simulink library "LIB_TF_G_112"  (Simulink 8.6)
settings: Solver=ode45  StartTime=0.0  StopTime=10.0  RelTol=1e-3
PreLoadFcn:
  | if exist('tl_preloadfcn','file'), tl_preloadfcn(gcs,402); end
PostLoadFcn:
  | if exist('tl_postloadfcn','file'), tl_postloadfcn(gcs,402); end
undefined symbols (not defined in the file): ddv, u2, u3
libraries: tllib x3
(part 1 of 4)
CloseFcn:
  | if exist('tl_closefcn','file'), tl_closefcn(gcs); end
settings Model: TLRevision=402  Creator=cedric.sauvage  LastModifiedBy=audrey.vache

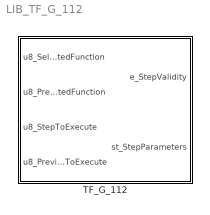
== system LIB_TF_G_112 ==
  TF_G_112 : Subsystem  TreatAsAtomicUnit=on

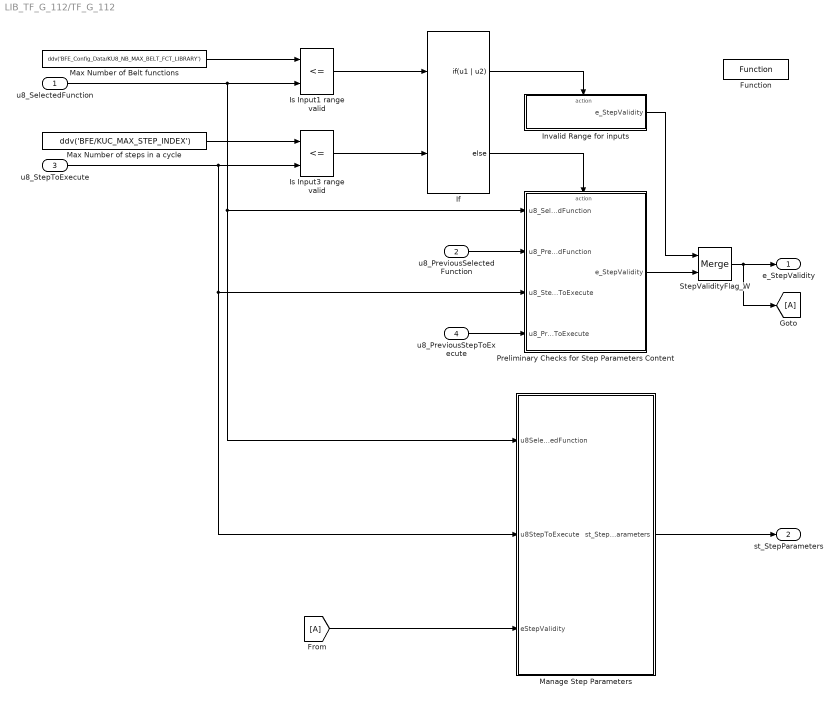
== system LIB_TF_G_112/TF_G_112 ==
  u8_SelectedFunction : Inport
  u8_PreviousSelectedFunction : Inport  Port=2
  u8_StepToExecute : Inport  Port=3
  u8_PreviousStepToExecute : Inport  Port=4
  Function : tllib/Function  data={'stepfunctionname','M_StepPreprocessing','stepfunctionclass','STATIC_FCN_ASR4','date',736467.70272937499}  displayString=FUNCTION
  If : If  NumInputs=2  IfExpression=u1 | u2
  Invalid Range for inputs : Subsystem  TreatAsAtomicUnit=on
  Is Input1 range valid : RelationalOperator  Operator=<=  OutDataTypeStr=boolean  mask(TL_RelationalOperator){data={'date',735951.66829449078}}
      settings: DeleteFcn=if exist('delete_tlblock','file')==2,delete_tlblock(gcbh);end  NameChangeFcn=if exist('rename_tlblock','file')==2,rename_tlblock(gcbh);end  OpenFcn=if exist('tl_open_blockdlg','file')==2,tl_open_blockdlg(gcbh);else,open_system(gcbh,'parameter');end
      mask Help: eval(['if exist(''tl_online_help'',''file'') == 2, tl_online_help(''Topic'',''TL_RelationalOperator''),else, web([''jar:file:///'',matlabroot,''/help/toolbox/simulink/help.jar!/slref/' lower(get_param(gcbh,'Blocktype')) '.html''], ''-helpbrowser''),end'])
      mask Display: plot([-0.05, 1.05, NaN, -0.05, 1.05],[.01, .01, NaN, .99, .99])
  Is Input3 range valid : RelationalOperator  Operator=<=  OutDataTypeStr=boolean  mask(TL_RelationalOperator){data={'date',735951.66829423606}}
      settings: DeleteFcn=if exist('delete_tlblock','file')==2,delete_tlblock(gcbh);end  NameChangeFcn=if exist('rename_tlblock','file')==2,rename_tlblock(gcbh);end  OpenFcn=if exist('tl_open_blockdlg','file')==2,tl_open_blockdlg(gcbh);else,open_system(gcbh,'parameter');end
      mask Help: eval(['if exist(''tl_online_help'',''file'') == 2, tl_online_help(''Topic'',''TL_RelationalOperator''),else, web([''jar:file:///'',matlabroot,''/help/toolbox/simulink/help.jar!/slref/' lower(get_param(gcbh,'Blocktype')) '.html''], ''-helpbrowser''),end'])
      mask Display: plot([-0.05, 1.05, NaN, -0.05, 1.05],[.01, .01, NaN, .99, .99])
  Manage Step Parameters : Subsystem  TreatAsAtomicUnit=on
  Max Number of Belt functions : Constant  Value=ddv('BFE_Config_Data/KU8_NB_MAX_BELT_FCT_LIBRARY')  mask(TL_Constant){data={'output',{'variable','BFE_Config_Data/KU8_NB_MAX_BELT_FCT_LIBRARY'},'date',735951.66825344902}}
      settings: CopyFcn=if exist('tl_reset_reviewflag','file')==2,tl_reset_reviewflag(gcbh);end  DeleteFcn=if exist('delete_tlblock','file')==2,delete_tlblock(gcbh);end  NameChangeFcn=if exist('rename_tlblock','file')==2,rename_tlblock(gcbh);end  OpenFcn=if exist('tl_open_blockdlg','file')==2,tl_open_blockdlg(gcbh);else,open_system(gcbh,'parameter');end
      mask Help: eval(['if exist(''tl_online_help'',''file'') == 2, tl_online_help(''Topic'',''TL_Constant''),else, web([''jar:file:///'',matlabroot,''/help/toolbox/simulink/help.jar!/slref/' lower(get_param(gcbh,'Blocktype')) '.html''], ''-helpbrowser''),end'])
      mask Display: plot([-0.05, 1.05, NaN, -0.05, 1.05],[.01, .01, NaN, .99, .99])
  Max Number of steps in a cycle : Constant  Value=ddv('BFE/KUC_MAX_STEP_INDEX')  mask(TL_Constant){data={'output',{'variable','BFE/KUC_MAX_STEP_INDEX'},'date',735951.66825306718}}
      settings: CopyFcn=if exist('tl_reset_reviewflag','file')==2,tl_reset_reviewflag(gcbh);end  DeleteFcn=if exist('delete_tlblock','file')==2,delete_tlblock(gcbh);end  NameChangeFcn=if exist('rename_tlblock','file')==2,rename_tlblock(gcbh);end  OpenFcn=if exist('tl_open_blockdlg','file')==2,tl_open_blockdlg(gcbh);else,open_system(gcbh,'parameter');end
      mask Help: eval(['if exist(''tl_online_help'',''file'') == 2, tl_online_help(''Topic'',''TL_Constant''),else, web([''jar:file:///'',matlabroot,''/help/toolbox/simulink/help.jar!/slref/' lower(get_param(gcbh,'Blocktype')) '.html''], ''-helpbrowser''),end'])
      mask Display: plot([-0.05, 1.05, NaN, -0.05, 1.05],[.01, .01, NaN, .99, .99])
  Preliminary Checks for Step Parameters Content : Subsystem  TreatAsAtomicUnit=on
  StepValidityFlag_W : Merge  InitialOutput=0  mask(TL_Merge){data={'logdata',{'maxnumvals',2500,'loggingmode',1},'output',{'name','eStepValidity','type','UInt8','inheritscaling',0},'date',735951.66823748848}}
      settings: CopyFcn=if exist('tl_reset_reviewflag','file')==2,tl_reset_reviewflag(gcbh);end  DeleteFcn=if exist('delete_tlblock','file')==2,delete_tlblock(gcbh);end  NameChangeFcn=if exist('rename_tlblock','file')==2,rename_tlblock(gcbh);end  OpenFcn=if exist('tl_open_blockdlg','file')==2,tl_open_blockdlg(gcbh);else,open_system(gcbh,'parameter');end
      mask Help: eval(['if exist(''tl_online_help'',''file'') == 2, tl_online_help(''Topic'',''TL_Merge''),else, web([''jar:file:///'',matlabroot,''/help/toolbox/simulink/help.jar!/slref/' lower(get_param(gcbh,'Blocktype')) '.html''], ''-helpbrowser''),end'])
      mask Display: plot([-0.05, 1.05, NaN, -0.05, 1.05],[.01, .01, NaN, .99, .99])
  e_StepValidity : Outport
  st_StepParameters : Outport  Port=2  OutDataTypeStr=Bus: stStepParameters
  wires:
  u8_SelectedFunction/1 -> Is Input1 range valid/2, Preliminary Checks for Step Parameters Content/1(u8_SelectedFunction), Manage Step Parameters/1(u8SelectedFunction)
  Max Number of Belt functions/1 -> Is Input1 range valid/1
  Max Number of steps in a cycle/1 -> Is Input3 range valid/1
  u8_StepToExecute/1 -> Is Input3 range valid/2, Preliminary Checks for Step Parameters Content/3(u8_StepToExecute), Manage Step Parameters/2(u8StepToExecute)
  If/1 -> Invalid Range for inputs/Action
  Is Input1 range valid/1 -> If/1
  Is Input3 range valid/1 -> If/2
  If/2 -> Preliminary Checks for Step Parameters Content/Action
  u8_PreviousSelectedFunction/1 -> Preliminary Checks for Step Parameters Content/2(u8_PreviousSelectedFunction)
  u8_PreviousStepToExecute/1 -> Preliminary Checks for Step Parameters Content/4(u8_PreviousStepToExecute)
  Preliminary Checks for Step Parameters Content/1(e_StepValidity) -> StepValidityFlag_W/2
  Invalid Range for inputs/1(e_StepValidity) -> StepValidityFlag_W/1
  StepValidityFlag_W/1 -> e_StepValidity/1, [A]
  Manage Step Parameters/1(st_StepParameters) -> st_StepParameters/1
  [A] -> Manage Step Parameters/3(eStepValidity)

== system LIB_TF_G_112/TF_G_112/Invalid Range for inputs ==
  note: COVERS: DES_TF_G_915
      | COVERS: DES_TF_G_916
      | COVERS: DES_TF_G_922
      | COVERS: DES_TF_G_923
  Action Port : ActionPort
  Invalid Step Key Value : Constant  Value=ddv('Internal_Interfaces/Enumerated_values/Step_Validity/KE_INVALID_STEP')  mask(TL_Constant){data={'output',{'variable','Internal_Interfaces/Enumerated_values/Step_Validity/KE_INVALID_STEP'},'date',735951.66829484957}}
      settings: CopyFcn=if exist('tl_reset_reviewflag','file')==2,tl_reset_reviewflag(gcbh);end  DeleteFcn=if exist('delete_tlblock','file')==2,delete_tlblock(gcbh);end  NameChangeFcn=if exist('rename_tlblock','file')==2,rename_tlblock(gcbh);end  OpenFcn=if exist('tl_open_blockdlg','file')==2,tl_open_blockdlg(gcbh);else,open_system(gcbh,'parameter');end
      mask Help: eval(['if exist(''tl_online_help'',''file'') == 2, tl_online_help(''Topic'',''TL_Constant''),else, web([''jar:file:///'',matlabroot,''/help/toolbox/simulink/help.jar!/slref/' lower(get_param(gcbh,'Blocktype')) '.html''], ''-helpbrowser''),end'])
      mask Display: plot([-0.05, 1.05, NaN, -0.05, 1.05],[.01, .01, NaN, .99, .99])
  e_StepValidity : Outport  InitialOutput=0
  wires:
  Invalid Step Key Value/1 -> e_StepValidity/1

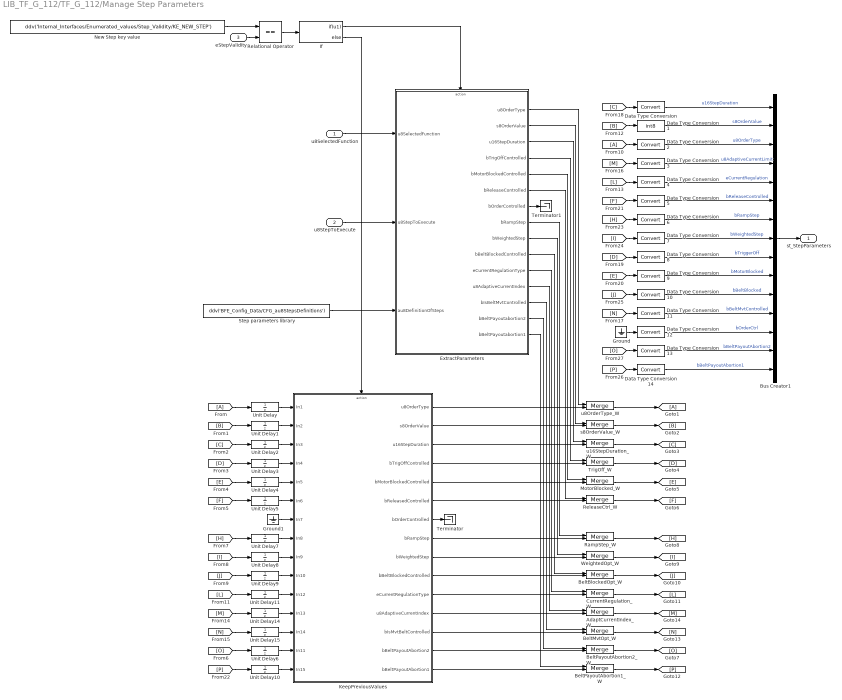
== system LIB_TF_G_112/TF_G_112/Manage Step Parameters ==
  u8SelectedFunction : Inport
  u8StepToExecute : Inport  Port=2
  eStepValidity : Inport  Port=3
  AdaptCurrentIndex_W : Merge  RequirementInfo={} %GIDa_e2928cb5_e14c_431e_87bc_c0c42f6fb32a  InitialOutput=ddv('Internal_Interfaces/stStepParameters/Components/u8AdaptCurrentLimit')  mask(TL_Merge){data={'logdata',{'loggingmode',1},'output',{'variable','Internal_Interfaces/stStepParameters/Components/u8AdaptCurrentLimit','inheritscaling',0},'date',735951.66829396994}}
      settings: CopyFcn=if exist('tl_reset_reviewflag','file')==2,tl_reset_reviewflag(gcbh);end  DeleteFcn=if exist('delete_tlblock','file')==2,delete_tlblock(gcbh);end  NameChangeFcn=if exist('rename_tlblock','file')==2,rename_tlblock(gcbh);end  OpenFcn=if exist('tl_open_blockdlg','file')==2,tl_open_blockdlg(gcbh);else,open_system(gcbh,'parameter');end
      mask Help: eval(['if exist(''tl_online_help'',''file'') == 2, tl_online_help(''Topic'',''TL_Merge''),else, web([''jar:file:///'',matlabroot,''/help/toolbox/simulink/help.jar!/slref/' lower(get_param(gcbh,'Blocktype')) '.html''], ''-helpbrowser''),end'])
      mask Display: plot([-0.05, 1.05, NaN, -0.05, 1.05],[.01, .01, NaN, .99, .99])
  BeltBlockedOpt_W : Merge  RequirementInfo={} %GIDa_0720534a_6e37_423d_8805_9648979410e2  InitialOutput=ddv('Internal_Interfaces/stStepParameters/Components/bBeltBlocked')  mask(TL_Merge){data={'logdata',{'loggingmode',1},'output',{'variable','Internal_Interfaces/stStepParameters/Components/bBeltBlocked','inheritscaling',0},'date',735951.66829357634}}
      settings: CopyFcn=if exist('tl_reset_reviewflag','file')==2,tl_reset_reviewflag(gcbh);end  DeleteFcn=if exist('delete_tlblock','file')==2,delete_tlblock(gcbh);end  NameChangeFcn=if exist('rename_tlblock','file')==2,rename_tlblock(gcbh);end  OpenFcn=if exist('tl_open_blockdlg','file')==2,tl_open_blockdlg(gcbh);else,open_system(gcbh,'parameter');end
      mask Help: eval(['if exist(''tl_online_help'',''file'') == 2, tl_online_help(''Topic'',''TL_Merge''),else, web([''jar:file:///'',matlabroot,''/help/toolbox/simulink/help.jar!/slref/' lower(get_param(gcbh,'Blocktype')) '.html''], ''-helpbrowser''),end'])
      mask Display: plot([-0.05, 1.05, NaN, -0.05, 1.05],[.01, .01, NaN, .99, .99])
  BeltMvtOpt_W : Merge  RequirementInfo={} %GIDa_23d3dad0_6239_4fa2_ab83_c69ad9dd92c5  InitialOutput=ddv('Internal_Interfaces/stStepParameters/Components/bBeltMvtDetection')  mask(TL_Merge){data={'logdata',{'loggingmode',1},'output',{'variable','Internal_Interfaces/stStepParameters/Components/bBeltMvtDetection','inheritscaling',0},'date',735951.66829317133}}
      settings: CopyFcn=if exist('tl_reset_reviewflag','file')==2,tl_reset_reviewflag(gcbh);end  DeleteFcn=if exist('delete_tlblock','file')==2,delete_tlblock(gcbh);end  NameChangeFcn=if exist('rename_tlblock','file')==2,rename_tlblock(gcbh);end  OpenFcn=if exist('tl_open_blockdlg','file')==2,tl_open_blockdlg(gcbh);else,open_system(gcbh,'parameter');end
      mask Help: eval(['if exist(''tl_online_help'',''file'') == 2, tl_online_help(''Topic'',''TL_Merge''),else, web([''jar:file:///'',matlabroot,''/help/toolbox/simulink/help.jar!/slref/' lower(get_param(gcbh,'Blocktype')) '.html''], ''-helpbrowser''),end'])
      mask Display: plot([-0.05, 1.05, NaN, -0.05, 1.05],[.01, .01, NaN, .99, .99])
  BeltPayoutAbortion1_W : Merge  RequirementInfo={} %GIDa_36c1306a_9619_4e1f_b53e_761d8c217ca4  InitialOutput=ddv('Internal_Interfaces/stStepParameters/Components/bBeltPayoutAbortion1')  mask(TL_Merge){data={'logdata',{'loggingmode',1},'output',{'variable','Internal_Interfaces/stStepParameters/Components/bBeltPayoutAbortion1','inheritscaling',0},'date',735951.66829277773}}
      settings: CopyFcn=if exist('tl_reset_reviewflag','file')==2,tl_reset_reviewflag(gcbh);end  DeleteFcn=if exist('delete_tlblock','file')==2,delete_tlblock(gcbh);end  NameChangeFcn=if exist('rename_tlblock','file')==2,rename_tlblock(gcbh);end  OpenFcn=if exist('tl_open_blockdlg','file')==2,tl_open_blockdlg(gcbh);else,open_system(gcbh,'parameter');end
      mask Help: eval(['if exist(''tl_online_help'',''file'') == 2, tl_online_help(''Topic'',''TL_Merge''),else, web([''jar:file:///'',matlabroot,''/help/toolbox/simulink/help.jar!/slref/' lower(get_param(gcbh,'Blocktype')) '.html''], ''-helpbrowser''),end'])
      mask Display: plot([-0.05, 1.05, NaN, -0.05, 1.05],[.01, .01, NaN, .99, .99])
  BeltPayoutAbortion2_W : Merge  RequirementInfo={} %GIDa_2edb20a6_a96c_4b43_add7_9deceefb659e  InitialOutput=ddv('Internal_Interfaces/stStepParameters/Components/bBeltPayoutAbortion2')  mask(TL_Merge){data={'logdata',{'loggingmode',1},'output',{'variable','Internal_Interfaces/stStepParameters/Components/bBeltPayoutAbortion2','inheritscaling',0},'date',735951.66829237272}}
      settings: CopyFcn=if exist('tl_reset_reviewflag','file')==2,tl_reset_reviewflag(gcbh);end  DeleteFcn=if exist('delete_tlblock','file')==2,delete_tlblock(gcbh);end  NameChangeFcn=if exist('rename_tlblock','file')==2,rename_tlblock(gcbh);end  OpenFcn=if exist('tl_open_blockdlg','file')==2,tl_open_blockdlg(gcbh);else,open_system(gcbh,'parameter');end
      mask Help: eval(['if exist(''tl_online_help'',''file'') == 2, tl_online_help(''Topic'',''TL_Merge''),else, web([''jar:file:///'',matlabroot,''/help/toolbox/simulink/help.jar!/slref/' lower(get_param(gcbh,'Blocktype')) '.html''], ''-helpbrowser''),end'])
      mask Display: plot([-0.05, 1.05, NaN, -0.05, 1.05],[.01, .01, NaN, .99, .99])
  Bus Creator1 : BusCreator  Inputs=15  OutDataTypeStr=Bus: stStepParameters
  CurrentRegulation_W : Merge  RequirementInfo={} %GIDa_a269fd5e_34b6_4587_839a_90c1f7d79006  InitialOutput=ddv('Internal_Interfaces/stStepParameters/Components/eCurrentRegulation')  mask(TL_Merge){data={'logdata',{'loggingmode',1},'output',{'variable','Internal_Interfaces/stStepParameters/Components/eCurrentRegulation','inheritscaling',0},'date',735951.66829194443}}
      settings: CopyFcn=if exist('tl_reset_reviewflag','file')==2,tl_reset_reviewflag(gcbh);end  DeleteFcn=if exist('delete_tlblock','file')==2,delete_tlblock(gcbh);end  NameChangeFcn=if exist('rename_tlblock','file')==2,rename_tlblock(gcbh);end  OpenFcn=if exist('tl_open_blockdlg','file')==2,tl_open_blockdlg(gcbh);else,open_system(gcbh,'parameter');end
      mask Help: eval(['if exist(''tl_online_help'',''file'') == 2, tl_online_help(''Topic'',''TL_Merge''),else, web([''jar:file:///'',matlabroot,''/help/toolbox/simulink/help.jar!/slref/' lower(get_param(gcbh,'Blocktype')) '.html''], ''-helpbrowser''),end'])
      mask Display: plot([-0.05, 1.05, NaN, -0.05, 1.05],[.01, .01, NaN, .99, .99])
  Data Type Conversion{,2..14} (14 alike) : DataTypeConversion
  Data Type Conversion1 : DataTypeConversion  OutDataTypeStr=int8
  ExtractParameters : Subsystem  RequirementInfo={} %GIDa_f8518a03_50c3_4128_a0d7_e66c9cadc317  TreatAsAtomicUnit=on
  Ground : Ground
  Ground1 : Ground
  If : If  IfExpression=u1
  KeepPreviousValues : Subsystem  RequirementInfo={} %GIDa_d99f78ca_cceb_45f0_b7aa_f1ab4b729ade  TreatAsAtomicUnit=on
  MotorBlocked_W : Merge  RequirementInfo={} %GIDa_09fb6a5e_7fa5_4304_8d3b_5ec2db5a55d7  InitialOutput=ddv('Internal_Interfaces/stStepParameters/Components/bMotorBlocked')  mask(TL_Merge){data={'logdata',{'loggingmode',1},'output',{'variable','Internal_Interfaces/stStepParameters/Components/bMotorBlocked','inheritscaling',0},'date',735951.66826525459}}
      settings: CopyFcn=if exist('tl_reset_reviewflag','file')==2,tl_reset_reviewflag(gcbh);end  DeleteFcn=if exist('delete_tlblock','file')==2,delete_tlblock(gcbh);end  NameChangeFcn=if exist('rename_tlblock','file')==2,rename_tlblock(gcbh);end  OpenFcn=if exist('tl_open_blockdlg','file')==2,tl_open_blockdlg(gcbh);else,open_system(gcbh,'parameter');end
      mask Help: eval(['if exist(''tl_online_help'',''file'') == 2, tl_online_help(''Topic'',''TL_Merge''),else, web([''jar:file:///'',matlabroot,''/help/toolbox/simulink/help.jar!/slref/' lower(get_param(gcbh,'Blocktype')) '.html''], ''-helpbrowser''),end'])
      mask Display: plot([-0.05, 1.05, NaN, -0.05, 1.05],[.01, .01, NaN, .99, .99])
  New Step key value : Constant  Value=ddv('Internal_Interfaces/Enumerated_values/Step_Validity/KE_NEW_STEP')  mask(TL_Constant){data={'output',{'variable','Internal_Interfaces/Enumerated_values/Step_Validity/KE_NEW_STEP'},'date',735951.66826484958}}
      settings: CopyFcn=if exist('tl_reset_reviewflag','file')==2,tl_reset_reviewflag(gcbh);end  DeleteFcn=if exist('delete_tlblock','file')==2,delete_tlblock(gcbh);end  NameChangeFcn=if exist('rename_tlblock','file')==2,rename_tlblock(gcbh);end  OpenFcn=if exist('tl_open_blockdlg','file')==2,tl_open_blockdlg(gcbh);else,open_system(gcbh,'parameter');end
      mask Help: eval(['if exist(''tl_online_help'',''file'') == 2, tl_online_help(''Topic'',''TL_Constant''),else, web([''jar:file:///'',matlabroot,''/help/toolbox/simulink/help.jar!/slref/' lower(get_param(gcbh,'Blocktype')) '.html''], ''-helpbrowser''),end'])
      mask Display: plot([-0.05, 1.05, NaN, -0.05, 1.05],[.01, .01, NaN, .99, .99])
  RampStep_W : Merge  RequirementInfo={} %GIDa_445c0878_ff8b_484e_8dd9_1f96a46135b1  InitialOutput=ddv('Internal_Interfaces/stStepParameters/Components/bRampStep')  mask(TL_Merge){data={'logdata',{'loggingmode',1},'output',{'variable','Internal_Interfaces/stStepParameters/Components/bRampStep','inheritscaling',0},'date',735951.66826444445}}
      settings: CopyFcn=if exist('tl_reset_reviewflag','file')==2,tl_reset_reviewflag(gcbh);end  DeleteFcn=if exist('delete_tlblock','file')==2,delete_tlblock(gcbh);end  NameChangeFcn=if exist('rename_tlblock','file')==2,rename_tlblock(gcbh);end  OpenFcn=if exist('tl_open_blockdlg','file')==2,tl_open_blockdlg(gcbh);else,open_system(gcbh,'parameter');end
      mask Help: eval(['if exist(''tl_online_help'',''file'') == 2, tl_online_help(''Topic'',''TL_Merge''),else, web([''jar:file:///'',matlabroot,''/help/toolbox/simulink/help.jar!/slref/' lower(get_param(gcbh,'Blocktype')) '.html''], ''-helpbrowser''),end'])
      mask Display: plot([-0.05, 1.05, NaN, -0.05, 1.05],[.01, .01, NaN, .99, .99])
  Relational Operator : RelationalOperator  Operator===  OutDataTypeStr=boolean  mask(TL_RelationalOperator){data={'date',735951.66826406249}}
      settings: DeleteFcn=if exist('delete_tlblock','file')==2,delete_tlblock(gcbh);end  NameChangeFcn=if exist('rename_tlblock','file')==2,rename_tlblock(gcbh);end  OpenFcn=if exist('tl_open_blockdlg','file')==2,tl_open_blockdlg(gcbh);else,open_system(gcbh,'parameter');end
      mask Help: eval(['if exist(''tl_online_help'',''file'') == 2, tl_online_help(''Topic'',''TL_RelationalOperator''),else, web([''jar:file:///'',matlabroot,''/help/toolbox/simulink/help.jar!/slref/' lower(get_param(gcbh,'Blocktype')) '.html''], ''-helpbrowser''),end'])
      mask Display: plot([-0.05, 1.05, NaN, -0.05, 1.05],[.01, .01, NaN, .99, .99])
  ReleaseCtrl_W : Merge  RequirementInfo={} %GIDa_7b701f30_aaf9_4e9e_a908_de5abfd09ea2  InitialOutput=ddv('Internal_Interfaces/stStepParameters/Components/bReleaseControlled')  mask(TL_Merge){data={'logdata',{'loggingmode',1},'output',{'variable','Internal_Interfaces/stStepParameters/Components/bReleaseControlled','inheritscaling',0},'date',735951.66826378473}}
      settings: CopyFcn=if exist('tl_reset_reviewflag','file')==2,tl_reset_reviewflag(gcbh);end  DeleteFcn=if exist('delete_tlblock','file')==2,delete_tlblock(gcbh);end  NameChangeFcn=if exist('rename_tlblock','file')==2,rename_tlblock(gcbh);end  OpenFcn=if exist('tl_open_blockdlg','file')==2,tl_open_blockdlg(gcbh);else,open_system(gcbh,'parameter');end
      mask Help: eval(['if exist(''tl_online_help'',''file'') == 2, tl_online_help(''Topic'',''TL_Merge''),else, web([''jar:file:///'',matlabroot,''/help/toolbox/simulink/help.jar!/slref/' lower(get_param(gcbh,'Blocktype')) '.html''], ''-helpbrowser''),end'])
      mask Display: plot([-0.05, 1.05, NaN, -0.05, 1.05],[.01, .01, NaN, .99, .99])
  Step parameters library : Constant  RequirementInfo={} %GIDa_701f29de_2d44_4d45_a297_c60af8fddfb1  Value=ddv('BFE_Config_Data/CFG_au8StepsDefinitions')  OutDataTypeStr=uint8  SampleTime=-1  mask(TL_Constant){data={'output',{'variable','BFE_Config_Data/CFG_au8StepsDefinitions'},'date',735951.66826340277}}
      settings: CopyFcn=if exist('tl_reset_reviewflag','file')==2,tl_reset_reviewflag(gcbh);end  DeleteFcn=if exist('delete_tlblock','file')==2,delete_tlblock(gcbh);end  NameChangeFcn=if exist('rename_tlblock','file')==2,rename_tlblock(gcbh);end  OpenFcn=if exist('tl_open_blockdlg','file')==2,tl_open_blockdlg(gcbh);else,open_system(gcbh,'parameter');end
      mask Help: eval(['if exist(''tl_online_help'',''file'') == 2, tl_online_help(''Topic'',''TL_Constant''),else, web([''jar:file:///'',matlabroot,''/help/toolbox/simulink/help.jar!/slref/' lower(get_param(gcbh,'Blocktype')) '.html''], ''-helpbrowser''),end'])
      mask Display: plot([-0.05, 1.05, NaN, -0.05, 1.05],[.01, .01, NaN, .99, .99])
  Terminator : Terminator
  Terminator1 : Terminator
  TrigOff_W : Merge  RequirementInfo={} %GIDa_825e8226_2cb9_4a51_a74d_7c94c7d3f7a5  InitialOutput=ddv('Internal_Interfaces/stStepParameters/Components/bTriggerOff')  mask(TL_Merge){data={'logdata',{'loggingmode',1},'output',{'variable','Internal_Interfaces/stStepParameters/Components/bTriggerOff','inheritscaling',0},'date',735951.66826290509}}
      settings: CopyFcn=if exist('tl_reset_reviewflag','file')==2,tl_reset_reviewflag(gcbh);end  DeleteFcn=if exist('delete_tlblock','file')==2,delete_tlblock(gcbh);end  NameChangeFcn=if exist('rename_tlblock','file')==2,rename_tlblock(gcbh);end  OpenFcn=if exist('tl_open_blockdlg','file')==2,tl_open_blockdlg(gcbh);else,open_system(gcbh,'parameter');end
      mask Help: eval(['if exist(''tl_online_help'',''file'') == 2, tl_online_help(''Topic'',''TL_Merge''),else, web([''jar:file:///'',matlabroot,''/help/toolbox/simulink/help.jar!/slref/' lower(get_param(gcbh,'Blocktype')) '.html''], ''-helpbrowser''),end'])
      mask Display: plot([-0.05, 1.05, NaN, -0.05, 1.05],[.01, .01, NaN, .99, .99])
  Unit Delay : UnitDelay  RequirementInfo={} %GIDa_6a8b625f_d9a6_4840_a588_d31e7d4b66fc  InitialCondition=7  SampleTime=-1  mask(TL_UnitDelay){data={'output',{'inheritscaling',1},'state',{'name','u8PrevOrderType','type','UInt8'},'date',735951.6682624768}}
      settings: CopyFcn=if exist('tl_reset_reviewflag','file')==2,tl_reset_reviewflag(gcbh);end  DeleteFcn=if exist('delete_tlblock','file')==2,delete_tlblock(gcbh);end  NameChangeFcn=if exist('rename_tlblock','file')==2,rename_tlblock(gcbh);end  OpenFcn=if exist('tl_open_blockdlg','file')==2,tl_open_blockdlg(gcbh);else,open_system(gcbh,'parameter');end
      mask Help: eval(['if exist(''tl_online_help'',''file'') == 2, tl_online_help(''Topic'',''TL_UnitDelay''),else, web([''jar:file:///'',matlabroot,''/help/toolbox/simulink/help.jar!/slref/' lower(get_param(gcbh,'Blocktype')) '.html''], ''-helpbrowser''),end'])
      mask Display: plot([-0.05, 1.05, NaN, -0.05, 1.05],[.01, .01, NaN, .99, .99])
  Unit Delay1 : UnitDelay  RequirementInfo={} %GIDa_3b60a22d_522f_464a_8320_3179146dea59  SampleTime=-1  mask(TL_UnitDelay){data={'output',{'inheritscaling',1},'state',{'name','s8PrevOrderValue','type','Int8'},'date',735951.66826194443}}
      settings: CopyFcn=if exist('tl_reset_reviewflag','file')==2,tl_reset_reviewflag(gcbh);end  DeleteFcn=if exist('delete_tlblock','file')==2,delete_tlblock(gcbh);end  NameChangeFcn=if exist('rename_tlblock','file')==2,rename_tlblock(gcbh);end  OpenFcn=if exist('tl_open_blockdlg','file')==2,tl_open_blockdlg(gcbh);else,open_system(gcbh,'parameter');end
      mask Help: eval(['if exist(''tl_online_help'',''file'') == 2, tl_online_help(''Topic'',''TL_UnitDelay''),else, web([''jar:file:///'',matlabroot,''/help/toolbox/simulink/help.jar!/slref/' lower(get_param(gcbh,'Blocktype')) '.html''], ''-helpbrowser''),end'])
      mask Display: plot([-0.05, 1.05, NaN, -0.05, 1.05],[.01, .01, NaN, .99, .99])
  Unit Delay10 : UnitDelay  RequirementInfo={} %GIDa_bcf95e16_89c3_42bc_ad91_cd19da001677  SampleTime=-1  mask(TL_UnitDelay){data={'output',{'inheritscaling',1},'state',{'name','bPrevBeltPayoutAbortion1'},'date',735951.66826143523}}
      settings: CopyFcn=if exist('tl_reset_reviewflag','file')==2,tl_reset_reviewflag(gcbh);end  DeleteFcn=if exist('delete_tlblock','file')==2,delete_tlblock(gcbh);end  NameChangeFcn=if exist('rename_tlblock','file')==2,rename_tlblock(gcbh);end  OpenFcn=if exist('tl_open_blockdlg','file')==2,tl_open_blockdlg(gcbh);else,open_system(gcbh,'parameter');end
      mask Help: eval(['if exist(''tl_online_help'',''file'') == 2, tl_online_help(''Topic'',''TL_UnitDelay''),else, web([''jar:file:///'',matlabroot,''/help/toolbox/simulink/help.jar!/slref/' lower(get_param(gcbh,'Blocktype')) '.html''], ''-helpbrowser''),end'])
      mask Display: plot([-0.05, 1.05, NaN, -0.05, 1.05],[.01, .01, NaN, .99, .99])
  Unit Delay11 : UnitDelay  RequirementInfo={} %GIDa_955c5a76_56d7_4fc9_870f_ec532b393a1a  SampleTime=-1  mask(TL_UnitDelay){data={'output',{'inheritscaling',1},'state',{'name','ePrevCurrentRegulationType'},'date',735951.66826090275}}
      settings: CopyFcn=if exist('tl_reset_reviewflag','file')==2,tl_reset_reviewflag(gcbh);end  DeleteFcn=if exist('delete_tlblock','file')==2,delete_tlblock(gcbh);end  NameChangeFcn=if exist('rename_tlblock','file')==2,rename_tlblock(gcbh);end  OpenFcn=if exist('tl_open_blockdlg','file')==2,tl_open_blockdlg(gcbh);else,open_system(gcbh,'parameter');end
      mask Help: eval(['if exist(''tl_online_help'',''file'') == 2, tl_online_help(''Topic'',''TL_UnitDelay''),else, web([''jar:file:///'',matlabroot,''/help/toolbox/simulink/help.jar!/slref/' lower(get_param(gcbh,'Blocktype')) '.html''], ''-helpbrowser''),end'])
      mask Display: plot([-0.05, 1.05, NaN, -0.05, 1.05],[.01, .01, NaN, .99, .99])
  Unit Delay14 : UnitDelay  RequirementInfo={} %GIDa_2c9f7313_0ff7_43a0_8e65_d7c9234dfdf6  SampleTime=-1  mask(TL_UnitDelay){data={'output',{'inheritscaling',1},'state',{'name','u8PrevCurrentIntPoint'},'date',735951.66826037038}}
      settings: CopyFcn=if exist('tl_reset_reviewflag','file')==2,tl_reset_reviewflag(gcbh);end  DeleteFcn=if exist('delete_tlblock','file')==2,delete_tlblock(gcbh);end  NameChangeFcn=if exist('rename_tlblock','file')==2,rename_tlblock(gcbh);end  OpenFcn=if exist('tl_open_blockdlg','file')==2,tl_open_blockdlg(gcbh);else,open_system(gcbh,'parameter');end
      mask Help: eval(['if exist(''tl_online_help'',''file'') == 2, tl_online_help(''Topic'',''TL_UnitDelay''),else, web([''jar:file:///'',matlabroot,''/help/toolbox/simulink/help.jar!/slref/' lower(get_param(gcbh,'Blocktype')) '.html''], ''-helpbrowser''),end'])
      mask Display: plot([-0.05, 1.05, NaN, -0.05, 1.05],[.01, .01, NaN, .99, .99])
  Unit Delay15 : UnitDelay  RequirementInfo={} %GIDa_55062164_f727_4870_9779_1a44e0735a6b  SampleTime=-1  mask(TL_UnitDelay){data={'output',{'inheritscaling',1},'state',{'name','bPrevBeltMvtFlg'},'date',735951.66825983801}}
      settings: CopyFcn=if exist('tl_reset_reviewflag','file')==2,tl_reset_reviewflag(gcbh);end  DeleteFcn=if exist('delete_tlblock','file')==2,delete_tlblock(gcbh);end  NameChangeFcn=if exist('rename_tlblock','file')==2,rename_tlblock(gcbh);end  OpenFcn=if exist('tl_open_blockdlg','file')==2,tl_open_blockdlg(gcbh);else,open_system(gcbh,'parameter');end
      mask Help: eval(['if exist(''tl_online_help'',''file'') == 2, tl_online_help(''Topic'',''TL_UnitDelay''),else, web([''jar:file:///'',matlabroot,''/help/toolbox/simulink/help.jar!/slref/' lower(get_param(gcbh,'Blocktype')) '.html''], ''-helpbrowser''),end'])
      mask Display: plot([-0.05, 1.05, NaN, -0.05, 1.05],[.01, .01, NaN, .99, .99])
  Unit Delay2 : UnitDelay  RequirementInfo={} %GIDa_46c8b873_30ec_40e9_ab3f_c62f0a32147c  SampleTime=-1  mask(TL_UnitDelay){data={'output',{'inheritscaling',1},'state',{'name','u16PrevStepDuration'},'date',735951.66825931717}}
      settings: CopyFcn=if exist('tl_reset_reviewflag','file')==2,tl_reset_reviewflag(gcbh);end  DeleteFcn=if exist('delete_tlblock','file')==2,delete_tlblock(gcbh);end  NameChangeFcn=if exist('rename_tlblock','file')==2,rename_tlblock(gcbh);end  OpenFcn=if exist('tl_open_blockdlg','file')==2,tl_open_blockdlg(gcbh);else,open_system(gcbh,'parameter');end
      mask Help: eval(['if exist(''tl_online_help'',''file'') == 2, tl_online_help(''Topic'',''TL_UnitDelay''),else, web([''jar:file:///'',matlabroot,''/help/toolbox/simulink/help.jar!/slref/' lower(get_param(gcbh,'Blocktype')) '.html''], ''-helpbrowser''),end'])
      mask Display: plot([-0.05, 1.05, NaN, -0.05, 1.05],[.01, .01, NaN, .99, .99])
  Unit Delay3 : UnitDelay  RequirementInfo={} %GIDa_4a163035_7b42_4ba8_9fe8_2325d4e00bc0  SampleTime=-1  mask(TL_UnitDelay){data={'output',{'inheritscaling',1},'state',{'name','bPrevTriggOffFlg'},'date',735951.66825879633}}
      settings: CopyFcn=if exist('tl_reset_reviewflag','file')==2,tl_reset_reviewflag(gcbh);end  DeleteFcn=if exist('delete_tlblock','file')==2,delete_tlblock(gcbh);end  NameChangeFcn=if exist('rename_tlblock','file')==2,rename_tlblock(gcbh);end  OpenFcn=if exist('tl_open_blockdlg','file')==2,tl_open_blockdlg(gcbh);else,open_system(gcbh,'parameter');end
      mask Help: eval(['if exist(''tl_online_help'',''file'') == 2, tl_online_help(''Topic'',''TL_UnitDelay''),else, web([''jar:file:///'',matlabroot,''/help/toolbox/simulink/help.jar!/slref/' lower(get_param(gcbh,'Blocktype')) '.html''], ''-helpbrowser''),end'])
      mask Display: plot([-0.05, 1.05, NaN, -0.05, 1.05],[.01, .01, NaN, .99, .99])
  Unit Delay4 : UnitDelay  RequirementInfo={} %GIDa_16ac9b19_c12f_41a7_9a03_56f1c61ef794  SampleTime=-1  mask(TL_UnitDelay){data={'output',{'inheritscaling',1},'state',{'name','bPrevMotorBlockedFlg'},'date',735951.66825825232}}
      settings: CopyFcn=if exist('tl_reset_reviewflag','file')==2,tl_reset_reviewflag(gcbh);end  DeleteFcn=if exist('delete_tlblock','file')==2,delete_tlblock(gcbh);end  NameChangeFcn=if exist('rename_tlblock','file')==2,rename_tlblock(gcbh);end  OpenFcn=if exist('tl_open_blockdlg','file')==2,tl_open_blockdlg(gcbh);else,open_system(gcbh,'parameter');end
      mask Help: eval(['if exist(''tl_online_help'',''file'') == 2, tl_online_help(''Topic'',''TL_UnitDelay''),else, web([''jar:file:///'',matlabroot,''/help/toolbox/simulink/help.jar!/slref/' lower(get_param(gcbh,'Blocktype')) '.html''], ''-helpbrowser''),end'])
      mask Display: plot([-0.05, 1.05, NaN, -0.05, 1.05],[.01, .01, NaN, .99, .99])
  Unit Delay5 : UnitDelay  RequirementInfo={} %GIDa_37b92a05_b534_4ec4_9d10_a1e6507e7de6  SampleTime=-1  mask(TL_UnitDelay){data={'output',{'inheritscaling',1},'state',{'name','bPrevRelCtrlFlg'},'date',735951.66825773148}}
      settings: CopyFcn=if exist('tl_reset_reviewflag','file')==2,tl_reset_reviewflag(gcbh);end  DeleteFcn=if exist('delete_tlblock','file')==2,delete_tlblock(gcbh);end  NameChangeFcn=if exist('rename_tlblock','file')==2,rename_tlblock(gcbh);end  OpenFcn=if exist('tl_open_blockdlg','file')==2,tl_open_blockdlg(gcbh);else,open_system(gcbh,'parameter');end
      mask Help: eval(['if exist(''tl_online_help'',''file'') == 2, tl_online_help(''Topic'',''TL_UnitDelay''),else, web([''jar:file:///'',matlabroot,''/help/toolbox/simulink/help.jar!/slref/' lower(get_param(gcbh,'Blocktype')) '.html''], ''-helpbrowser''),end'])
      mask Display: plot([-0.05, 1.05, NaN, -0.05, 1.05],[.01, .01, NaN, .99, .99])
  Unit Delay6 : UnitDelay  RequirementInfo={} %GIDa_a4f43ca0_4394_4154_98b6_a71f1ee0790a  SampleTime=-1  mask(TL_UnitDelay){data={'output',{'inheritscaling',1},'state',{'name','bPrevBeltPayoutAbortion2'},'date',735951.66825721064}}
      settings: CopyFcn=if exist('tl_reset_reviewflag','file')==2,tl_reset_reviewflag(gcbh);end  DeleteFcn=if exist('delete_tlblock','file')==2,delete_tlblock(gcbh);end  NameChangeFcn=if exist('rename_tlblock','file')==2,rename_tlblock(gcbh);end  OpenFcn=if exist('tl_open_blockdlg','file')==2,tl_open_blockdlg(gcbh);else,open_system(gcbh,'parameter');end
      mask Help: eval(['if exist(''tl_online_help'',''file'') == 2, tl_online_help(''Topic'',''TL_UnitDelay''),else, web([''jar:file:///'',matlabroot,''/help/toolbox/simulink/help.jar!/slref/' lower(get_param(gcbh,'Blocktype')) '.html''], ''-helpbrowser''),end'])
      mask Display: plot([-0.05, 1.05, NaN, -0.05, 1.05],[.01, .01, NaN, .99, .99])
  Unit Delay7 : UnitDelay  RequirementInfo={} %GIDa_e5a95ff3_fc02_49a5_aa2f_390ce4a6a578  SampleTime=-1  mask(TL_UnitDelay){data={'output',{'inheritscaling',1},'state',{'name','bPrevRampFlg'},'date',735951.66825668979}}
      settings: CopyFcn=if exist('tl_reset_reviewflag','file')==2,tl_reset_reviewflag(gcbh);end  DeleteFcn=if exist('delete_tlblock','file')==2,delete_tlblock(gcbh);end  NameChangeFcn=if exist('rename_tlblock','file')==2,rename_tlblock(gcbh);end  OpenFcn=if exist('tl_open_blockdlg','file')==2,tl_open_blockdlg(gcbh);else,open_system(gcbh,'parameter');end
      mask Help: eval(['if exist(''tl_online_help'',''file'') == 2, tl_online_help(''Topic'',''TL_UnitDelay''),else, web([''jar:file:///'',matlabroot,''/help/toolbox/simulink/help.jar!/slref/' lower(get_param(gcbh,'Blocktype')) '.html''], ''-helpbrowser''),end'])
      mask Display: plot([-0.05, 1.05, NaN, -0.05, 1.05],[.01, .01, NaN, .99, .99])
  Unit Delay8 : UnitDelay  RequirementInfo={} %GIDa_f7672656_0a25_4e21_bcec_4dc5f0f39bde  SampleTime=-1  mask(TL_UnitDelay){data={'output',{'inheritscaling',1},'state',{'name','bPrevWeightedFlg'},'date',735951.66825615743}}
      settings: CopyFcn=if exist('tl_reset_reviewflag','file')==2,tl_reset_reviewflag(gcbh);end  DeleteFcn=if exist('delete_tlblock','file')==2,delete_tlblock(gcbh);end  NameChangeFcn=if exist('rename_tlblock','file')==2,rename_tlblock(gcbh);end  OpenFcn=if exist('tl_open_blockdlg','file')==2,tl_open_blockdlg(gcbh);else,open_system(gcbh,'parameter');end
      mask Help: eval(['if exist(''tl_online_help'',''file'') == 2, tl_online_help(''Topic'',''TL_UnitDelay''),else, web([''jar:file:///'',matlabroot,''/help/toolbox/simulink/help.jar!/slref/' lower(get_param(gcbh,'Blocktype')) '.html''], ''-helpbrowser''),end'])
      mask Display: plot([-0.05, 1.05, NaN, -0.05, 1.05],[.01, .01, NaN, .99, .99])
  Unit Delay9 : UnitDelay  RequirementInfo={} %GIDa_ffd523ab_2bb6_4658_b154_fd46d981c1bf  SampleTime=-1  mask(TL_UnitDelay){data={'output',{'inheritscaling',1},'state',{'name','bPrevBeltBlockedFlg'},'date',735951.66825562494}}
      settings: CopyFcn=if exist('tl_reset_reviewflag','file')==2,tl_reset_reviewflag(gcbh);end  DeleteFcn=if exist('delete_tlblock','file')==2,delete_tlblock(gcbh);end  NameChangeFcn=if exist('rename_tlblock','file')==2,rename_tlblock(gcbh);end  OpenFcn=if exist('tl_open_blockdlg','file')==2,tl_open_blockdlg(gcbh);else,open_system(gcbh,'parameter');end
      mask Help: eval(['if exist(''tl_online_help'',''file'') == 2, tl_online_help(''Topic'',''TL_UnitDelay''),else, web([''jar:file:///'',matlabroot,''/help/toolbox/simulink/help.jar!/slref/' lower(get_param(gcbh,'Blocktype')) '.html''], ''-helpbrowser''),end'])
      mask Display: plot([-0.05, 1.05, NaN, -0.05, 1.05],[.01, .01, NaN, .99, .99])
  WeightedOpt_W : Merge  RequirementInfo={} %GIDa_77d438e3_c130_4039_9d97_7a4272cb0cdf  InitialOutput=ddv('Internal_Interfaces/stStepParameters/Components/bWeightedStep')  mask(TL_Merge){data={'logdata',{'loggingmode',1},'output',{'variable','Internal_Interfaces/stStepParameters/Components/bWeightedStep','inheritscaling',0},'date',735951.66825509258}}
      settings: CopyFcn=if exist('tl_reset_reviewflag','file')==2,tl_reset_reviewflag(gcbh);end  DeleteFcn=if exist('delete_tlblock','file')==2,delete_tlblock(gcbh);end  NameChangeFcn=if exist('rename_tlblock','file')==2,rename_tlblock(gcbh);end  OpenFcn=if exist('tl_open_blockdlg','file')==2,tl_open_blockdlg(gcbh);else,open_system(gcbh,'parameter');end
      mask Help: eval(['if exist(''tl_online_help'',''file'') == 2, tl_online_help(''Topic'',''TL_Merge''),else, web([''jar:file:///'',matlabroot,''/help/toolbox/simulink/help.jar!/slref/' lower(get_param(gcbh,'Blocktype')) '.html''], ''-helpbrowser''),end'])
      mask Display: plot([-0.05, 1.05, NaN, -0.05, 1.05],[.01, .01, NaN, .99, .99])
  s8OrderValue_W : Merge  RequirementInfo={} %GIDa_9146a6a1_c3dd_43fd_b49d_8a72e354e92f  InitialOutput=ddv('Internal_Interfaces/stStepParameters/Components/s8OrderValue')  mask(TL_Merge){data={'logdata',{'loggingmode',1},'output',{'variable','Internal_Interfaces/stStepParameters/Components/s8OrderValue','inheritscaling',0},'date',735951.66825469909}}
      settings: CopyFcn=if exist('tl_reset_reviewflag','file')==2,tl_reset_reviewflag(gcbh);end  DeleteFcn=if exist('delete_tlblock','file')==2,delete_tlblock(gcbh);end  NameChangeFcn=if exist('rename_tlblock','file')==2,rename_tlblock(gcbh);end  OpenFcn=if exist('tl_open_blockdlg','file')==2,tl_open_blockdlg(gcbh);else,open_system(gcbh,'parameter');end
      mask Help: eval(['if exist(''tl_online_help'',''file'') == 2, tl_online_help(''Topic'',''TL_Merge''),else, web([''jar:file:///'',matlabroot,''/help/toolbox/simulink/help.jar!/slref/' lower(get_param(gcbh,'Blocktype')) '.html''], ''-helpbrowser''),end'])
      mask Display: plot([-0.05, 1.05, NaN, -0.05, 1.05],[.01, .01, NaN, .99, .99])
  u16StepDuration_W : Merge  RequirementInfo={} %GIDa_ffc47c3a_3ae9_4d19_bffb_b2a8ca4d2a69  InitialOutput=ddv('Internal_Interfaces/stStepParameters/Components/u16StepDuration')  mask(TL_Merge){data={'logdata',{'loggingmode',1},'output',{'variable','Internal_Interfaces/stStepParameters/Components/u16StepDuration','inheritscaling',0},'date',735951.66825430561}}
      settings: CopyFcn=if exist('tl_reset_reviewflag','file')==2,tl_reset_reviewflag(gcbh);end  DeleteFcn=if exist('delete_tlblock','file')==2,delete_tlblock(gcbh);end  NameChangeFcn=if exist('rename_tlblock','file')==2,rename_tlblock(gcbh);end  OpenFcn=if exist('tl_open_blockdlg','file')==2,tl_open_blockdlg(gcbh);else,open_system(gcbh,'parameter');end
      mask Help: eval(['if exist(''tl_online_help'',''file'') == 2, tl_online_help(''Topic'',''TL_Merge''),else, web([''jar:file:///'',matlabroot,''/help/toolbox/simulink/help.jar!/slref/' lower(get_param(gcbh,'Blocktype')) '.html''], ''-helpbrowser''),end'])
      mask Display: plot([-0.05, 1.05, NaN, -0.05, 1.05],[.01, .01, NaN, .99, .99])
  u8OrderType_W : Merge  RequirementInfo={} %GIDa_5609f3d3_6e01_47c8_ab18_eeebdcb5af63  InitialOutput=ddv('Internal_Interfaces/stStepParameters/Components/u8OrderType')  mask(TL_Merge){data={'logdata',{'loggingmode',1},'output',{'variable','Internal_Interfaces/stStepParameters/Components/u8OrderType','inheritscaling',0},'date',735951.66825388884}}
      settings: CopyFcn=if exist('tl_reset_reviewflag','file')==2,tl_reset_reviewflag(gcbh);end  DeleteFcn=if exist('delete_tlblock','file')==2,delete_tlblock(gcbh);end  NameChangeFcn=if exist('rename_tlblock','file')==2,rename_tlblock(gcbh);end  OpenFcn=if exist('tl_open_blockdlg','file')==2,tl_open_blockdlg(gcbh);else,open_system(gcbh,'parameter');end
      mask Help: eval(['if exist(''tl_online_help'',''file'') == 2, tl_online_help(''Topic'',''TL_Merge''),else, web([''jar:file:///'',matlabroot,''/help/toolbox/simulink/help.jar!/slref/' lower(get_param(gcbh,'Blocktype')) '.html''], ''-helpbrowser''),end'])
      mask Display: plot([-0.05, 1.05, NaN, -0.05, 1.05],[.01, .01, NaN, .99, .99])
  st_StepParameters : Outport
  wires:
  New Step key value/1 -> Relational Operator/1
  eStepValidity/1 -> Relational Operator/2
  Relational Operator/1 -> If/1
  If/2 -> KeepPreviousValues/Action
  u8OrderType_W/1 -> [A]
  s8OrderValue_W/1 -> [B]
  u16StepDuration_W/1 -> [C]
  TrigOff_W/1 -> [D]
  MotorBlocked_W/1 -> [E]
  ReleaseCtrl_W/1 -> [F]
  RampStep_W/1 -> [H]
  BeltBlockedOpt_W/1 -> [J]
  CurrentRegulation_W/1 -> [L]
  AdaptCurrentIndex_W/1 -> [M]
  BeltMvtOpt_W/1 -> [N]
  ExtractParameters/1(u8OrderType) -> u8OrderType_W/1
  ExtractParameters/2(s8OrderValue) -> s8OrderValue_W/1
  ExtractParameters/3(u16StepDuration) -> u16StepDuration_W/1
  ExtractParameters/4(bTrigOffControlled) -> TrigOff_W/1
  ExtractParameters/5(bMotorBlockedControlled) -> MotorBlocked_W/1
  ExtractParameters/6(bReleaseControlled) -> ReleaseCtrl_W/1
  ExtractParameters/8(bRampStep) -> RampStep_W/1
  ExtractParameters/9(bWeightedStep) -> WeightedOpt_W/1
  ExtractParameters/10(bBeltBlockedControlled) -> BeltBlockedOpt_W/1
  ExtractParameters/11(eCurrentRegulationType) -> CurrentRegulation_W/1
  ExtractParameters/12(u8AdaptiveCurrentIndex) -> AdaptCurrentIndex_W/1
  ExtractParameters/13(bIsBeltMvtControlled) -> BeltMvtOpt_W/1
  KeepPreviousValues/1(u8OrderType) -> u8OrderType_W/2
  KeepPreviousValues/2(s8OrderValue) -> s8OrderValue_W/2
  KeepPreviousValues/3(u16StepDuration) -> u16StepDuration_W/2
  KeepPreviousValues/4(bTrigOffControlled) -> TrigOff_W/2
  KeepPreviousValues/5(bMotorBlockedControlled) -> MotorBlocked_W/2
  KeepPreviousValues/6(bReleasedControlled) -> ReleaseCtrl_W/2
  KeepPreviousValues/8(bRampStep) -> RampStep_W/2
  KeepPreviousValues/9(bWeightedStep) -> WeightedOpt_W/2
  KeepPreviousValues/10(bBeltBlockedControlled) -> BeltBlockedOpt_W/2
  KeepPreviousValues/11(eCurrentRegulationType) -> CurrentRegulation_W/2
  KeepPreviousValues/12(u8AdaptiveCurrentIndex) -> AdaptCurrentIndex_W/2
  KeepPreviousValues/13(bIsMvtBeltControlled) -> BeltMvtOpt_W/2
  Unit Delay/1 -> KeepPreviousValues/1(In1)
  [A] -> Unit Delay/1
  Unit Delay1/1 -> KeepPreviousValues/2(In2)
  [B] -> Unit Delay1/1
  [C] -> Unit Delay2/1
  Unit Delay2/1 -> KeepPreviousValues/3(In3)
  Unit Delay3/1 -> KeepPreviousValues/4(In4)
  [D] -> Unit Delay3/1
  Unit Delay4/1 -> KeepPreviousValues/5(In5)
  [E] -> Unit Delay4/1
  [F] -> Unit Delay5/1
  Unit Delay5/1 -> KeepPreviousValues/6(In6)
  Unit Delay7/1 -> KeepPreviousValues/8(In8)
  [H] -> Unit Delay7/1
  [I] -> Unit Delay8/1
  Unit Delay8/1 -> KeepPreviousValues/9(In9)
  Unit Delay9/1 -> KeepPreviousValues/10(In10)
  [J] -> Unit Delay9/1
  [L] -> Unit Delay11/1
  Unit Delay11/1 -> KeepPreviousValues/11(In12)
  [M] -> Unit Delay14/1
  Unit Delay14/1 -> KeepPreviousValues/12(In13)
  Unit Delay15/1 -> KeepPreviousValues/13(In14)
  [N] -> Unit Delay15/1
  If/1 -> ExtractParameters/Action
  Step parameters library/1 -> ExtractParameters/3(au8DefinitionOfSteps)
  Bus Creator1/1 -> st_StepParameters/1
  WeightedOpt_W/1 -> [I]
  [C] -> Data Type Conversion/1
  [B] -> Data Type Conversion1/1
  [A] -> Data Type Conversion2/1
  [M] -> Data Type Conversion3/1
  [L] -> Data Type Conversion4/1
  [F] -> Data Type Conversion5/1
  [H] -> Data Type Conversion6/1
  [I] -> Data Type Conversion7/1
  [D] -> Data Type Conversion8/1
  [E] -> Data Type Conversion9/1
  [J] -> Data Type Conversion10/1
  [N] -> Data Type Conversion11/1
  Ground/1 -> Data Type Conversion12/1
  Data Type Conversion/1 -> Bus Creator1/1  "u16StepDuration"
  Data Type Conversion1/1 -> Bus Creator1/2  "s8OrderValue"
  Data Type Conversion2/1 -> Bus Creator1/3  "u8OrderType"
  Data Type Conversion3/1 -> Bus Creator1/4  "u8AdaptiveCurrentLimit"
  Data Type Conversion4/1 -> Bus Creator1/5  "eCurrentRegulation"
  Data Type Conversion5/1 -> Bus Creator1/6  "bReleaseControlled"
  Data Type Conversion6/1 -> Bus Creator1/7  "bRampStep"
  Data Type Conversion7/1 -> Bus Creator1/8  "bWeightedStep"
  Data Type Conversion8/1 -> Bus Creator1/9  "bTriggerOff"
  Data Type Conversion9/1 -> Bus Creator1/10  "bMotorBlocked"
  Data Type Conversion10/1 -> Bus Creator1/11  "bBeltBlocked"
  Data Type Conversion11/1 -> Bus Creator1/12  "bBeltMvtControlled"
  Data Type Conversion12/1 -> Bus Creator1/13  "bOrderCtrl"
  Ground1/1 -> KeepPreviousValues/7(In7)
  KeepPreviousValues/7(bOrderControlled) -> Terminator/1
  ExtractParameters/7(bOrderControlled) -> Terminator1/1
  u8SelectedFunction/1 -> ExtractParameters/1(u8SelectedFunction)
  u8StepToExecute/1 -> ExtractParameters/2(u8StepToExecute)
  BeltPayoutAbortion2_W/1 -> [O]
  BeltPayoutAbortion1_W/1 -> [P]
  KeepPreviousValues/14(bBeltPayoutAbortion2) -> BeltPayoutAbortion2_W/2
  KeepPreviousValues/15(bBeltPayoutAbortion1) -> BeltPayoutAbortion1_W/2
  [O] -> Unit Delay6/1
  Unit Delay6/1 -> KeepPreviousValues/14(In11)
  [P] -> Unit Delay10/1
  Unit Delay10/1 -> KeepPreviousValues/15(In15)
  [O] -> Data Type Conversion13/1
  [P] -> Data Type Conversion14/1
  Data Type Conversion13/1 -> Bus Creator1/14  "bBeltPayoutAbortion2"
  Data Type Conversion14/1 -> Bus Creator1/15  "bBeltPayoutAbortion1"
  ExtractParameters/14(bBeltPayoutabortion2) -> BeltPayoutAbortion2_W/1
  ExtractParameters/15(bBeltPayoutabortion1) -> BeltPayoutAbortion1_W/1
